simulink model "SCR_SiLS2"  (R2021b)
settings: Solver=FixedStepDiscrete  StartTime=0.0  StopTime=inf  FixedStep=0.001  RelTol=1e-3
model workspace (MAT data in the model file):
  DataSet = []
  DebugLevel = 0
  GuiObj = 0
  GuiObjTemp = 0
  GuiPrefs.ColVis = [1 1 1 1 1 1 1 1 1 0]
  GuiPrefs.Mode = 0
  GuiPrefs.View = 1
  GuiPrefs.Hierarchy = 1
  GuiPrefs.BatchMode = 0
  GuiPrefs.ConsistentAccess = 0
  M1TargetParameters.TargetIp = '192.168.0.153'
  M1TargetParameters.M1ControllerName = 'M1Controller'
  M1TargetParameters.SwModuleName = 'SILS'
  M1TargetParameters.ApplPartition = 2
  M1TargetParameters.BasePriority = 30
  M1TargetParameters.CoreCategory = ''
  M1TargetParameters.DownlToM1Contr = 'on'
  M1TargetParameters.PermanentInstall = 'on'
  M1TargetParameters.DeviceOnM1 = 'Application path'
  M1TargetParameters.SendEOI = 'on'
  M1TargetParameters.ControllerUsr = 'M1'
  M1TargetParameters.ControllerPwd = 'bachmann'
  M1TargetParameters.ModDebugLevel = '0x0'
  NbrOfParams = 0
  NbrOfRem = 0
  save_DataSet = []
  save_NbrOfParams = 0
  save_NbrOfRem = 0
undefined symbols (not defined in the file or in its folder): AI_Test1, AO_Test1, NONOXR4, PLC_PRG, var1_INT16_LREAL_scalar_bus_200_mixed_aligned_out, X20I0Mat_typ, X20IOMat, X20IOSim
libraries: bur_blks x62, M1SWBlocks x11, simulink x1
(part 1 of 2)
CloseFcn:
  | ModelCloseCallback(gcs, 'FigureName', 'M1DownloadSettings');
  | ModelCloseCallback(gcs, 'FigureName', 'SourceInclusion');
settings Model: ExtModeSkipDownloadWhenConnect=on  Creator=gione  LastModifiedBy=gione
settings HardwareCC: ProdBitPerPointer=32  ProdBitPerSizeT=32  ProdBitPerPtrDiffT=32  ProdLargestAtomicInteger=Long  ProdWordSize=32  ProdLongLongMode=on  ProdHWDeviceType=Bachmann->Bachmann M1 Controller  TargetLargestAtomicInteger=Long  TargetLargestAtomicFloat=Float  TargetLongLongMode=on  TargetIntDivRoundTo=Zero  TargetEndianess=LittleEndian  TargetHWDeviceType=Bachmann->Bachmann M1 Controller  ProdEqTarget=off
settings RTWCC: Description=Bachmann M1 SW Module Creator  SystemTargetFile=m1target.tlc  TemplateMakefile=m1target.tmf  GenerateReport=on  LaunchReport=on
settings STFCustomTargetCC: SystemTargetFile=m1target.tlc
settings GRTTargetCC: TargetLangStandard=C89/C90 (ANSI)  ParMdlRefBuildCompliant=off  CompOptLevelCompliant=off  ConcurrentExecutionCompliant=off  CombineOutputUpdateFcns=off  MatFileLogging=off  CPPClassGenCompliant=off  GRTInterface=on  UseToolchainInfoCompliant=off  ExtMode=on  ExtModeMexFile=ext_m1target_comm  ExtModeMexArgs='192.168.0.153' 0 17725 'SILS' 'M1' 'bachmann'

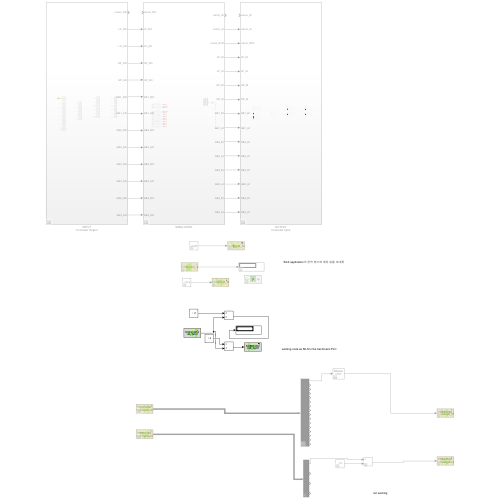
[thumbnail: Simulink's stored preview of the top-level diagram]
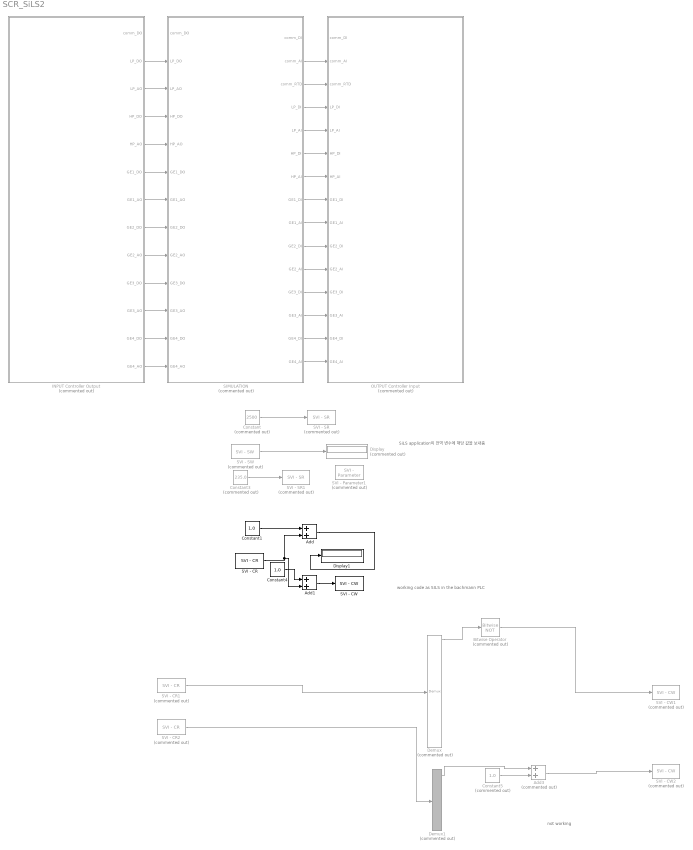
== system SCR_SiLS2 ==
  note: SiLS application의 전역 변수에 해당 값을 보내줌
  note: working code as SILS in the bachmann PLC
  note: not working
  Add : Sum
  Add1 : Sum
  Add3 : Sum  Commented=on
  Bitwise Operator : simulink/Logic and Bit Operations/Bitwise Operator  Commented=on  logicop=NOT  UseBitMask=off  BitMask=bin2dec('11011001')  BitMaskRealWorld=Stored Integer
  Constant : Constant  Commented=on  Value=2500
  Constant1 : Constant  Value=1.0
  Constant3 : Constant  Commented=on  Value=235.0
      settings: CopyFcn=CopyBlockEntries(gcs, gcb, 'Constant3');  DeleteFcn=RefreshFile(gcs, gcb, 1);  NameChangeFcn=RefreshFile(gcs, gcb, 0);
  Constant4 : Constant  Value=1.0
  Constant5 : Constant  Commented=on  Value=1.0
  Demux : Demux  Commented=on  Outputs=16  BusSelectionMode=on
  Demux1 : Demux  Commented=on  BusSelectionMode=on
  Display : Display  Commented=on
  Display1 : Display
  INPUT Controller Output : Subsystem  Commented=on
  OUTPUT Controller Input : Subsystem  Commented=on
  SIMULATION : Subsystem  Commented=on
  SVI - CR : M1SWBlocks/SVI Blocks/SVI - CR  Description=SVI client read block  svi_taskname=NONOXR4  svi_varname=.AI_Test1  svi_datatype=double  svi_retcodeoutput=off  svi_enablesettrigger=off  svi_settrigger=rising  svi_reconnect=off  svi_valdurlostconn=Last value  svi_valueinternal=567657567567  svi_sampletime=0.001  svi_simavailable=off  svi_roundtype=Zero
      settings: SourceProductName=Bachmann M1 Software
  SVI - CR1 : M1SWBlocks/SVI Blocks/SVI - CR  Description=SVI client read block  Commented=on  svi_taskname=NONOXR4  svi_varname=.IOSim/Comm/DI_0  svi_datatype=Bus: DO_Value  svi_retcodeoutput=off  svi_enablesettrigger=off  svi_settrigger=rising  svi_reconnect=off  svi_valdurlostconn=Last value  svi_valueinternal=567657567567  svi_sampletime=Ts_com  svi_simavailable=off  svi_roundtype=Zero
      settings: SourceProductName=Bachmann M1 Software
  SVI - CR2 : M1SWBlocks/SVI Blocks/SVI - CR  Description=SVI client read block  Commented=on  svi_taskname=NONOXR4  svi_varname=.IOSim/Comm/AO_0  svi_datatype=Bus: AO_Value  svi_retcodeoutput=off  svi_enablesettrigger=off  svi_settrigger=rising  svi_reconnect=off  svi_valdurlostconn=Last value  svi_valueinternal=567657567567  svi_sampletime=Ts_com  svi_simavailable=off  svi_roundtype=Zero
      settings: SourceProductName=Bachmann M1 Software
  SVI - CW : M1SWBlocks/SVI Blocks/SVI - CW  Description=SVI client write block  svi_taskname=NONOXR4  svi_varname=.AO_Test1  svi_datatype=double  svi_roundtype=Zero  svi_retcodeoutput=off  svi_enablesettrigger=off  svi_settrigger=rising  svi_reconnect=off  svi_simavailable=off
      settings: SourceProductName=Bachmann M1 Software
  SVI - CW1 : M1SWBlocks/SVI Blocks/SVI - CW  Description=SVI client write block  Commented=on  svi_taskname=NONOXR4  svi_varname='.IOSim/Comm/DI_0/Value0'  svi_datatype=boolean  svi_roundtype=Zero  svi_retcodeoutput=off  svi_enablesettrigger=off  svi_settrigger=rising  svi_reconnect=off  svi_simavailable=off
      settings: SourceProductName=Bachmann M1 Software
  SVI - CW2 : M1SWBlocks/SVI Blocks/SVI - CW  Description=SVI client write block  Commented=on  svi_taskname=NONOXR4  svi_varname='NONOXR4/.IOSim/Comm/AI_0/Value0'  svi_datatype=single  svi_roundtype=Zero  svi_retcodeoutput=off  svi_enablesettrigger=off  svi_settrigger=rising  svi_reconnect=off  svi_simavailable=off
      settings: SourceProductName=Bachmann M1 Software
  SVI - Parameter1 : M1SWBlocks/SVI Blocks/SVI - Parameter  Commented=on  svi_changeCount=1
      settings: SourceProductName=Bachmann M1 Software
  SVI - SR : M1SWBlocks/SVI Blocks/SVI - SR  Description=SVI server readonly block  Commented=on  svi_name=NONOXR4/AI_Test1  svi_modelname=off  svi_subsysname=off  svi_datatype=Inherit: auto  svi_alignment=4 bytes aligned  svi_roundtype=Nearest  svi_consistent=off  svi_simavailable=off
      settings: SourceProductName=Bachmann M1 Software
  SVI - SR1 : M1SWBlocks/SVI Blocks/SVI - SR  Description=SVI server readonly block  Commented=on  svi_name=NONOXR4/AI_Test1  svi_modelname=off  svi_subsysname=off  svi_datatype=Inherit: auto  svi_alignment=4 bytes aligned  svi_roundtype=Nearest  svi_consistent=off  svi_simavailable=off
      settings: SourceProductName=Bachmann M1 Software
  SVI - SW : M1SWBlocks/SVI Blocks/SVI - SW  Description=SVI server read/write block  Commented=on  svi_name=NONOXR4/AO_Test1  svi_modelname=off  svi_subsysname=off  svi_initvalue=0  svi_datatype=Inherit: Inherit via back propagation  svi_alignment=4 bytes aligned  svi_varremanent=off  svi_consistent=on  svi_sampletime=-1  svi_simavailable=off  svi_roundtype=Zero
      settings: SourceProductName=Bachmann M1 Software
  wires:
  Constant/1 -> SVI - SR/1
  SVI - SW/1 -> Display/1
  Constant1/1 -> Add/1
  SVI - CR/1 -> Add1/2, Add/2
  Add/1 -> Display1/1
  Constant3/1 -> SVI - SR1/1
  Constant4/1 -> Add1/1
  Add1/1 -> SVI - CW/1
  SIMULATION/15(GE4_AI) -> OUTPUT Controller Input/15(GE4_AI)
  SIMULATION/14(GE4_DI) -> OUTPUT Controller Input/14(GE4_DI)
  SIMULATION/11(GE2_AI) -> OUTPUT Controller Input/11(GE2_AI)
  SIMULATION/4(LP_DI) -> OUTPUT Controller Input/4(LP_DI)
  SIMULATION/5(LP_AI) -> OUTPUT Controller Input/5(LP_AI)
  INPUT Controller Output/9(GE2_AO) -> SIMULATION/9(GE2_AO)
  INPUT Controller Output/10(GE3_DO) -> SIMULATION/10(GE3_DO)
  INPUT Controller Output/7(GE1_AO) -> SIMULATION/7(GE1_AO)
  INPUT Controller Output/8(GE2_DO) -> SIMULATION/8(GE2_DO)
  INPUT Controller Output/6(GE1_DO) -> SIMULATION/6(GE1_DO)
  INPUT Controller Output/3(LP_AO) -> SIMULATION/3(LP_AO)
  INPUT Controller Output/4(HP_DO) -> SIMULATION/4(HP_DO)
  SIMULATION/2(comm_AI) -> OUTPUT Controller Input/2(comm_AI)
  SIMULATION/8(GE1_DI) -> OUTPUT Controller Input/8(GE1_DI)
  INPUT Controller Output/5(HP_AO) -> SIMULATION/5(HP_AO)
  INPUT Controller Output/2(LP_DO) -> SIMULATION/2(LP_DO)
  SIMULATION/6(HP_DI) -> OUTPUT Controller Input/6(HP_DI)
  SIMULATION/13(GE3_AI) -> OUTPUT Controller Input/13(GE3_AI)
  SIMULATION/9(GE1_AI) -> OUTPUT Controller Input/9(GE1_AI)
  SIMULATION/3(comm_RTD) -> OUTPUT Controller Input/3(comm_RTD)
  INPUT Controller Output/13(GE4_AO) -> SIMULATION/13(GE4_AO)
  INPUT Controller Output/12(GE4_DO) -> SIMULATION/12(GE4_DO)
  INPUT Controller Output/11(GE3_AO) -> SIMULATION/11(GE3_AO)
  SIMULATION/7(HP_AI) -> OUTPUT Controller Input/7(HP_AI)
  SIMULATION/12(GE3_DI) -> OUTPUT Controller Input/12(GE3_DI)
  SIMULATION/10(GE2_DI) -> OUTPUT Controller Input/10(GE2_DI)
  SVI - CR1/1 -> Demux/1
  Demux/1 -> Bitwise Operator/1
  SVI - CR2/1 -> Demux1/1
  Demux1/1 -> Add3/1
  Add3/1 -> SVI - CW2/1
  Bitwise Operator/1 -> SVI - CW1/1
  Constant5/1 -> Add3/2

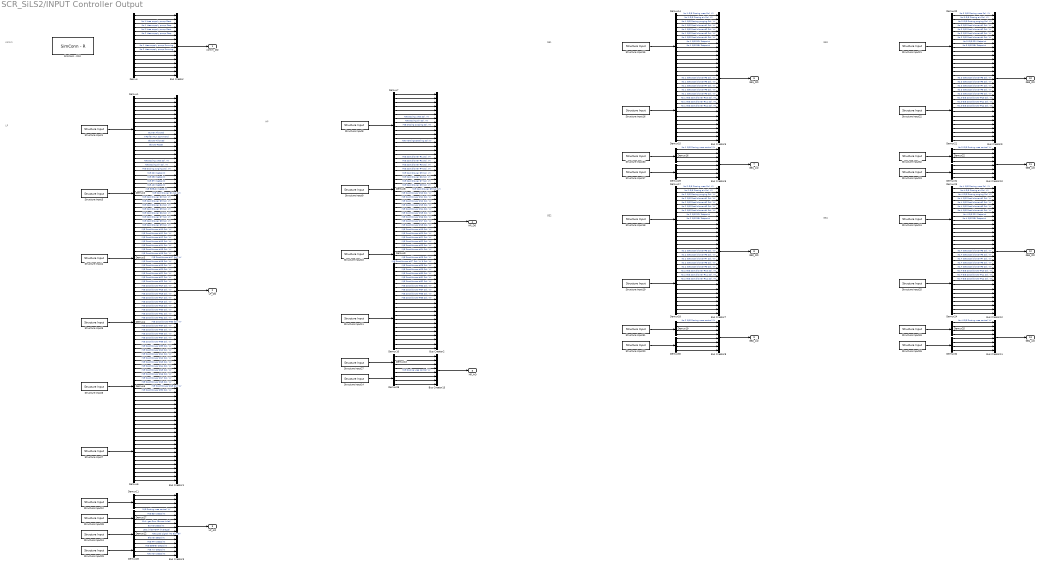
== system SCR_SiLS2/INPUT Controller Output ==
  note: comm
  note: LP
  note: HP
  note: GE1
  note: GE2
  note: GE3
  note: GE4
  Bus Creator : BusCreator  Inputs=16
  Bus Creator1 : BusCreator  Inputs=96
  Bus Creator{6,8,10..11,13} (5 alike) : BusCreator  Inputs=8
  Bus Creator{5,7,9,12} (4 alike) : BusCreator  Inputs=32
  Bus Creator2 : BusCreator  Inputs=64
  Bus Creator3 : BusCreator  Inputs=16
  Demux{,1..10,14..15,17..18,20..21,23..24} (19 alike) : Demux  Outputs=16
  Demux{11..13,16,19,22,25..32} (14 alike) : Demux
  SimConn - R10 : M1SWBlocks/SimConn Blocks/SimConn - R  connVarName=ConnVar  InswModuleName='NONOXR4'  swModuleName=PLC_DSRC  InvarName='.X20IOSim.Comm.DOF322[0].Value'  varName=PLC_PRG/var1_INT16_LREAL_scalar_bus_200_mixed_aligned_out  varDataType=Inherit: Inherit via back propagation  enRetOutput=on  enGetTrigger=off  getTrigger=rising  valDurLostConn=Zero  internalVal=0  DataDim=1  enSampTimMon=on  sampleTime=Ts_com
      settings: SourceProductName=Bachmann M1 Software
  Structure Input1 : bur_blks/Structure Input  Tag=GLOBAL BOOL X20IOSim.LP.DOF322[0].Value [0...15]  bur_var_name=X20IOSim.LP.DOF322[0].Value  bur_scope=GLOBAL  bur_struct_name=X20IOSim  bur_data_type=BOOL  bur_array_index=15  bur_data_type_num=8  bur_AS_string=X20IOSim : X20I0Mat_typ := (0); (**)  bur_struct_reference=X20I0Mat_typ.LP.DOF322(0).Value  bur_memory=standard
      settings: AttributesFormatString=%<Tag>  SourceProductName=B&R Automation Studio Toolbox
  Structure Input10 : bur_blks/Structure Input  Tag=GLOBAL BOOL X20IOSim.HP.DOF322[2].Value [0...15]  bur_var_name=X20IOSim.HP.DOF322[2].Value  bur_scope=GLOBAL  bur_struct_name=X20IOSim  bur_data_type=BOOL  bur_array_index=15  bur_data_type_num=8  bur_AS_string=X20IOSim : X20I0Mat_typ := (0); (**)  bur_struct_reference=X20I0Mat_typ.HP.DOF322(2).Value  bur_memory=standard
      settings: AttributesFormatString=%<Tag>  SourceProductName=B&R Automation Studio Toolbox
  Structure Input11 : bur_blks/Structure Input  Tag=GLOBAL BOOL X20IOSim.HP.DOF322[3].Value [0...15]  bur_var_name=X20IOSim.HP.DOF322[3].Value  bur_scope=GLOBAL  bur_struct_name=X20IOSim  bur_data_type=BOOL  bur_array_index=15  bur_data_type_num=8  bur_AS_string=X20IOSim : X20I0Mat_typ := (0); (**)  bur_struct_reference=X20I0Mat_typ.HP.DOF322(3).Value  bur_memory=standard
      settings: AttributesFormatString=%<Tag>  SourceProductName=B&R Automation Studio Toolbox
  Structure Input12 : bur_blks/Structure Input  Tag=GLOBAL REAL X20IOSim.LP.AO4622[0].Value [0...3]  bur_var_name=X20IOSim.LP.AO4622[0].Value  bur_scope=GLOBAL  bur_struct_name=X20IOSim  bur_data_type=REAL  bur_array_index=3  bur_data_type_num=1  bur_AS_string=X20IOSim : X20I0Mat_typ := (0); (**)  bur_struct_reference=X20I0Mat_typ.LP.AO4622(0).Value  bur_memory=standard
      settings: AttributesFormatString=%<Tag>  SourceProductName=B&R Automation Studio Toolbox
  Structure Input13 : bur_blks/Structure Input  Tag=GLOBAL REAL X20IOSim.LP.AO4622[2].Value [0...3]  bur_var_name=X20IOSim.LP.AO4622[2].Value  bur_scope=GLOBAL  bur_struct_name=X20IOSim  bur_data_type=REAL  bur_array_index=3  bur_data_type_num=1  bur_AS_string=X20IOSim : X20I0Mat_typ := (0); (**)  bur_struct_reference=X20I0Mat_typ.LP.AO4622(2).Value  bur_memory=standard
      settings: AttributesFormatString=%<Tag>  SourceProductName=B&R Automation Studio Toolbox
  Structure Input14 : bur_blks/Structure Input  Tag=GLOBAL REAL X20IOSim.HP.AO4622[1].Value [0...3]  bur_var_name=X20IOSim.HP.AO4622[1].Value  bur_scope=GLOBAL  bur_struct_name=X20IOSim  bur_data_type=REAL  bur_array_index=3  bur_data_type_num=1  bur_AS_string=X20IOSim : X20I0Mat_typ := (0); (**)  bur_struct_reference=X20I0Mat_typ.HP.AO4622(1).Value  bur_memory=standard
      settings: AttributesFormatString=%<Tag>  SourceProductName=B&R Automation Studio Toolbox
  Structure Input15 : bur_blks/Structure Input  Tag=GLOBAL BOOL X20IOSim.GE1.DOF322[0].Value [0...15]  bur_var_name=X20IOSim.GE1.DOF322[0].Value  bur_scope=GLOBAL  bur_struct_name=X20IOSim  bur_data_type=BOOL  bur_array_index=15  bur_data_type_num=8  bur_AS_string=X20IOSim : X20I0Mat_typ := (0); (**)  bur_struct_reference=X20I0Mat_typ.GE1.DOF322(0).Value  bur_memory=standard
      settings: AttributesFormatString=%<Tag>  SourceProductName=B&R Automation Studio Toolbox
  Structure Input16 : bur_blks/Structure Input  Tag=GLOBAL BOOL X20IOSim.GE1.DOF322[1].Value [0...15]  bur_var_name=X20IOSim.GE1.DOF322[1].Value  bur_scope=GLOBAL  bur_struct_name=X20IOSim  bur_data_type=BOOL  bur_array_index=15  bur_data_type_num=8  bur_AS_string=X20IOSim : X20I0Mat_typ := (0); (**)  bur_struct_reference=X20I0Mat_typ.GE1.DOF322(1).Value  bur_memory=standard
      settings: AttributesFormatString=%<Tag>  SourceProductName=B&R Automation Studio Toolbox
  Structure Input17 : bur_blks/Structure Input  Tag=GLOBAL REAL X20IOSim.GE1.AO4622[1].Value [0...3]  bur_var_name=X20IOSim.GE1.AO4622[1].Value  bur_scope=GLOBAL  bur_struct_name=X20IOSim  bur_data_type=REAL  bur_array_index=3  bur_data_type_num=1  bur_AS_string=X20IOSim : X20I0Mat_typ := (0); (**)  bur_struct_reference=X20I0Mat_typ.GE1.AO4622(1).Value  bur_memory=standard
      settings: AttributesFormatString=%<Tag>  SourceProductName=B&R Automation Studio Toolbox
  Structure Input18 : bur_blks/Structure Input  Tag=GLOBAL BOOL X20IOSim.GE2.DOF322[0].Value [0...15]  bur_var_name=X20IOSim.GE2.DOF322[0].Value  bur_scope=GLOBAL  bur_struct_name=X20IOSim  bur_data_type=BOOL  bur_array_index=15  bur_data_type_num=8  bur_AS_string=X20IOSim : X20I0Mat_typ := (0); (**)  bur_struct_reference=X20I0Mat_typ.GE2.DOF322(0).Value  bur_memory=standard
      settings: AttributesFormatString=%<Tag>  SourceProductName=B&R Automation Studio Toolbox
  Structure Input19 : bur_blks/Structure Input  Tag=GLOBAL BOOL X20IOSim.GE2.DOF322[1].Value [0...15]  bur_var_name=X20IOSim.GE2.DOF322[1].Value  bur_scope=GLOBAL  bur_struct_name=X20IOSim  bur_data_type=BOOL  bur_array_index=15  bur_data_type_num=8  bur_AS_string=X20IOSim : X20I0Mat_typ := (0); (**)  bur_struct_reference=X20I0Mat_typ.GE2.DOF322(1).Value  bur_memory=standard
      settings: AttributesFormatString=%<Tag>  SourceProductName=B&R Automation Studio Toolbox
  Structure Input20 : bur_blks/Structure Input  Tag=GLOBAL REAL X20IOSim.GE2.AO4622[1].Value [0...3]  bur_var_name=X20IOSim.GE2.AO4622[1].Value  bur_scope=GLOBAL  bur_struct_name=X20IOSim  bur_data_type=REAL  bur_array_index=3  bur_data_type_num=1  bur_AS_string=X20IOSim : X20I0Mat_typ := (0); (**)  bur_struct_reference=X20I0Mat_typ.GE2.AO4622(1).Value  bur_memory=standard
      settings: AttributesFormatString=%<Tag>  SourceProductName=B&R Automation Studio Toolbox
  Structure Input21 : bur_blks/Structure Input  Tag=GLOBAL BOOL X20IOSim.GE3.DOF322[0].Value [0...15]  bur_var_name=X20IOSim.GE3.DOF322[0].Value  bur_scope=GLOBAL  bur_struct_name=X20IOSim  bur_data_type=BOOL  bur_array_index=15  bur_data_type_num=8  bur_AS_string=X20IOSim : X20I0Mat_typ := (0); (**)  bur_struct_reference=X20I0Mat_typ.GE3.DOF322(0).Value  bur_memory=standard
      settings: AttributesFormatString=%<Tag>  SourceProductName=B&R Automation Studio Toolbox
  Structure Input22 : bur_blks/Structure Input  Tag=GLOBAL BOOL X20IOSim.GE3.DOF322[1].Value [0...15]  bur_var_name=X20IOSim.GE3.DOF322[1].Value  bur_scope=GLOBAL  bur_struct_name=X20IOSim  bur_data_type=BOOL  bur_array_index=15  bur_data_type_num=8  bur_AS_string=X20IOSim : X20I0Mat_typ := (0); (**)  bur_struct_reference=X20I0Mat_typ.GE3.DOF322(1).Value  bur_memory=standard
      settings: AttributesFormatString=%<Tag>  SourceProductName=B&R Automation Studio Toolbox
  Structure Input23 : bur_blks/Structure Input  Tag=GLOBAL REAL X20IOSim.GE3.AO4622[1].Value [0...3]  bur_var_name=X20IOSim.GE3.AO4622[1].Value  bur_scope=GLOBAL  bur_struct_name=X20IOSim  bur_data_type=REAL  bur_array_index=3  bur_data_type_num=1  bur_AS_string=X20IOSim : X20I0Mat_typ := (0); (**)  bur_struct_reference=X20I0Mat_typ.GE3.AO4622(1).Value  bur_memory=standard
      settings: AttributesFormatString=%<Tag>  SourceProductName=B&R Automation Studio Toolbox
  Structure Input24 : bur_blks/Structure Input  Tag=GLOBAL BOOL X20IOSim.GE4.DOF322[0].Value [0...15]  bur_var_name=X20IOSim.GE4.DOF322[0].Value  bur_scope=GLOBAL  bur_struct_name=X20IOSim  bur_data_type=BOOL  bur_array_index=15  bur_data_type_num=8  bur_AS_string=X20IOSim : X20I0Mat_typ := (0); (**)  bur_struct_reference=X20I0Mat_typ.GE4.DOF322(0).Value  bur_memory=standard
      settings: AttributesFormatString=%<Tag>  SourceProductName=B&R Automation Studio Toolbox
  Structure Input25 : bur_blks/Structure Input  Tag=GLOBAL BOOL X20IOSim.GE4.DOF322[1].Value [0...15]  bur_var_name=X20IOSim.GE4.DOF322[1].Value  bur_scope=GLOBAL  bur_struct_name=X20IOSim  bur_data_type=BOOL  bur_array_index=15  bur_data_type_num=8  bur_AS_string=X20IOSim : X20I0Mat_typ := (0); (**)  bur_struct_reference=X20I0Mat_typ.GE4.DOF322(1).Value  bur_memory=standard
      settings: AttributesFormatString=%<Tag>  SourceProductName=B&R Automation Studio Toolbox
  Structure Input26 : bur_blks/Structure Input  Tag=GLOBAL REAL X20IOSim.GE4.AO4622[1].Value [0...3]  bur_var_name=X20IOSim.GE4.AO4622[1].Value  bur_scope=GLOBAL  bur_struct_name=X20IOSim  bur_data_type=REAL  bur_array_index=3  bur_data_type_num=1  bur_AS_string=X20IOSim : X20I0Mat_typ := (0); (**)  bur_struct_reference=X20I0Mat_typ.GE4.AO4622(1).Value  bur_memory=standard
      settings: AttributesFormatString=%<Tag>  SourceProductName=B&R Automation Studio Toolbox
  Structure Input27 : bur_blks/Structure Input  Tag=GLOBAL REAL X20IOSim.HP.AO4622[0].Value [0...3]  bur_var_name=X20IOSim.HP.AO4622[0].Value  bur_scope=GLOBAL  bur_struct_name=X20IOSim  bur_data_type=REAL  bur_array_index=3  bur_data_type_num=1  bur_AS_string=X20IOSim : X20I0Mat_typ := (0); (**)  bur_struct_reference=X20I0Mat_typ.HP.AO4622(0).Value  bur_memory=standard
      settings: AttributesFormatString=%<Tag>  SourceProductName=B&R Automation Studio Toolbox
  Structure Input28 : bur_blks/Structure Input  Tag=GLOBAL REAL X20IOSim.LP.AO4622[1].Value [0...3]  bur_var_name=X20IOSim.LP.AO4622[1].Value  bur_scope=GLOBAL  bur_struct_name=X20IOSim  bur_data_type=REAL  bur_array_index=3  bur_data_type_num=1  bur_AS_string=X20IOSim : X20I0Mat_typ := (0); (**)  bur_struct_reference=X20I0Mat_typ.LP.AO4622(1).Value  bur_memory=standard
      settings: AttributesFormatString=%<Tag>  SourceProductName=B&R Automation Studio Toolbox
  Structure Input29 : bur_blks/Structure Input  Tag=GLOBAL REAL X20IOSim.LP.AO4622[3].Value [0...3]  bur_var_name=X20IOSim.LP.AO4622[3].Value  bur_scope=GLOBAL  bur_struct_name=X20IOSim  bur_data_type=REAL  bur_array_index=3  bur_data_type_num=1  bur_AS_string=X20IOSim : X20I0Mat_typ := (0); (**)  bur_struct_reference=X20I0Mat_typ.LP.AO4622(3).Value  bur_memory=standard
      settings: AttributesFormatString=%<Tag>  SourceProductName=B&R Automation Studio Toolbox
  Structure Input3 : bur_blks/Structure Input  Tag=GLOBAL BOOL X20IOSim.LP.DOF322[1].Value [0...15]  bur_var_name=X20IOSim.LP.DOF322[1].Value  bur_scope=GLOBAL  bur_struct_name=X20IOSim  bur_data_type=BOOL  bur_array_index=15  bur_data_type_num=8  bur_AS_string=X20IOSim : X20I0Mat_typ := (0); (**)  bur_struct_reference=X20I0Mat_typ.LP.DOF322(1).Value  bur_memory=standard
      settings: AttributesFormatString=%<Tag>  SourceProductName=B&R Automation Studio Toolbox
  Structure Input30 : bur_blks/Structure Input  Tag=GLOBAL REAL X20IOSim.GE1.AO4622[0].Value [0...3]  bur_var_name=X20IOSim.GE1.AO4622[0].Value  bur_scope=GLOBAL  bur_struct_name=X20IOSim  bur_data_type=REAL  bur_array_index=3  bur_data_type_num=1  bur_AS_string=X20IOSim : X20I0Mat_typ := (0); (**)  bur_struct_reference=X20I0Mat_typ.GE1.AO4622(0).Value  bur_memory=standard
      settings: AttributesFormatString=%<Tag>  SourceProductName=B&R Automation Studio Toolbox
  Structure Input31 : bur_blks/Structure Input  Tag=GLOBAL REAL X20IOSim.GE2.AO4622[0].Value [0...3]  bur_var_name=X20IOSim.GE2.AO4622[0].Value  bur_scope=GLOBAL  bur_struct_name=X20IOSim  bur_data_type=REAL  bur_array_index=3  bur_data_type_num=1  bur_AS_string=X20IOSim : X20I0Mat_typ := (0); (**)  bur_struct_reference=X20I0Mat_typ.GE2.AO4622(0).Value  bur_memory=standard
      settings: AttributesFormatString=%<Tag>  SourceProductName=B&R Automation Studio Toolbox
  Structure Input32 : bur_blks/Structure Input  Tag=GLOBAL REAL X20IOSim.GE3.AO4622[0].Value [0...3]  bur_var_name=X20IOSim.GE3.AO4622[0].Value  bur_scope=GLOBAL  bur_struct_name=X20IOSim  bur_data_type=REAL  bur_array_index=3  bur_data_type_num=1  bur_AS_string=X20IOSim : X20I0Mat_typ := (0); (**)  bur_struct_reference=X20I0Mat_typ.GE3.AO4622(0).Value  bur_memory=standard
      settings: AttributesFormatString=%<Tag>  SourceProductName=B&R Automation Studio Toolbox
  Structure Input33 : bur_blks/Structure Input  Tag=GLOBAL REAL X20IOSim.GE4.AO4622[0].Value [0...3]  bur_var_name=X20IOSim.GE4.AO4622[0].Value  bur_scope=GLOBAL  bur_struct_name=X20IOSim  bur_data_type=REAL  bur_array_index=3  bur_data_type_num=1  bur_AS_string=X20IOSim : X20I0Mat_typ := (0); (**)  bur_struct_reference=X20I0Mat_typ.GE4.AO4622(0).Value  bur_memory=standard
      settings: AttributesFormatString=%<Tag>  SourceProductName=B&R Automation Studio Toolbox
  Structure Input4 : bur_blks/Structure Input  Tag=GLOBAL BOOL X20IOSim.LP.DOF322[2].Value [0...15]  bur_var_name=X20IOSim.LP.DOF322[2].Value  bur_scope=GLOBAL  bur_struct_name=X20IOSim  bur_data_type=BOOL  bur_array_index=15  bur_data_type_num=8  bur_AS_string=X20IOSim : X20I0Mat_typ := (0); (**)  bur_struct_reference=X20I0Mat_typ.LP.DOF322(2).Value  bur_memory=standard
      settings: AttributesFormatString=%<Tag>  SourceProductName=B&R Automation Studio Toolbox
  Structure Input5 : bur_blks/Structure Input  Tag=GLOBAL BOOL X20IOSim.LP.DOF322[3].Value [0...15]  bur_var_name=X20IOSim.LP.DOF322[3].Value  bur_scope=GLOBAL  bur_struct_name=X20IOSim  bur_data_type=BOOL  bur_array_index=15  bur_data_type_num=8  bur_AS_string=X20IOSim : X20I0Mat_typ := (0); (**)  bur_struct_reference=X20I0Mat_typ.LP.DOF322(3).Value  bur_memory=standard
      settings: AttributesFormatString=%<Tag>  SourceProductName=B&R Automation Studio Toolbox
  Structure Input6 : bur_blks/Structure Input  Tag=GLOBAL BOOL X20IOSim.LP.DOF322[4].Value [0...15]  bur_var_name=X20IOSim.LP.DOF322[4].Value  bur_scope=GLOBAL  bur_struct_name=X20IOSim  bur_data_type=BOOL  bur_array_index=15  bur_data_type_num=8  bur_AS_string=X20IOSim : X20I0Mat_typ := (0); (**)  bur_struct_reference=X20I0Mat_typ.LP.DOF322(4).Value  bur_memory=standard
      settings: AttributesFormatString=%<Tag>  SourceProductName=B&R Automation Studio Toolbox
  Structure Input7 : bur_blks/Structure Input  Tag=GLOBAL BOOL X20IOSim.LP.DOF322[5].Value [0...15]  bur_var_name=X20IOSim.LP.DOF322[5].Value  bur_scope=GLOBAL  bur_struct_name=X20IOSim  bur_data_type=BOOL  bur_array_index=15  bur_data_type_num=8  bur_AS_string=X20IOSim : X20I0Mat_typ := (0); (**)  bur_struct_reference=X20I0Mat_typ.LP.DOF322(5).Value  bur_memory=standard
      settings: AttributesFormatString=%<Tag>  SourceProductName=B&R Automation Studio Toolbox
  Structure Input8 : bur_blks/Structure Input  Tag=GLOBAL BOOL X20IOSim.HP.DOF322[0].Value [0...15]  bur_var_name=X20IOSim.HP.DOF322[0].Value  bur_scope=GLOBAL  bur_struct_name=X20IOSim  bur_data_type=BOOL  bur_array_index=15  bur_data_type_num=8  bur_AS_string=X20IOSim : X20I0Mat_typ := (0); (**)  bur_struct_reference=X20I0Mat_typ.HP.DOF322(0).Value  bur_memory=standard
      settings: AttributesFormatString=%<Tag>  SourceProductName=B&R Automation Studio Toolbox
  Structure Input9 : bur_blks/Structure Input  Tag=GLOBAL BOOL X20IOSim.HP.DOF322[1].Value [0...15]  bur_var_name=X20IOSim.HP.DOF322[1].Value  bur_scope=GLOBAL  bur_struct_name=X20IOSim  bur_data_type=BOOL  bur_array_index=15  bur_data_type_num=8  bur_AS_string=X20IOSim : X20I0Mat_typ := (0); (**)  bur_struct_reference=X20I0Mat_typ.HP.DOF322(1).Value  bur_memory=standard
      settings: AttributesFormatString=%<Tag>  SourceProductName=B&R Automation Studio Toolbox
  comm_DO : Outport  VectorParamsAs1DForOutWhenUnconnected=off
  LP_DO : Outport  Port=2  VectorParamsAs1DForOutWhenUnconnected=off
  LP_AO : Outport  Port=3  VectorParamsAs1DForOutWhenUnconnected=off
  HP_DO : Outport  Port=4  VectorParamsAs1DForOutWhenUnconnected=off
  HP_AO : Outport  Port=5  VectorParamsAs1DForOutWhenUnconnected=off
  GE1_DO : Outport  Port=6  VectorParamsAs1DForOutWhenUnconnected=off
  GE1_AO : Outport  Port=7  VectorParamsAs1DForOutWhenUnconnected=off
  GE2_DO : Outport  Port=8  VectorParamsAs1DForOutWhenUnconnected=off
  GE2_AO : Outport  Port=9  VectorParamsAs1DForOutWhenUnconnected=off
  GE3_DO : Outport  Port=10  VectorParamsAs1DForOutWhenUnconnected=off
  GE3_AO : Outport  Port=11  VectorParamsAs1DForOutWhenUnconnected=off
  GE4_DO : Outport  Port=12  VectorParamsAs1DForOutWhenUnconnected=off
  GE4_AO : Outport  Port=13  VectorParamsAs1DForOutWhenUnconnected=off
  wires:
  Demux17/11 -> Bus Creator7/11
  Demux10/14 -> Bus Creator2/62
  Demux3/8 -> Bus Creator1/40  "M/E Soot blower #16 Sol. VV"
  Demux17/7 -> Bus Creator7/7  "No.2 G/E Soot blower #4 Sol. VV"
  Demux11/4 -> Bus Creator3/4
  Demux5/2 -> Bus Creator1/66  "M/E Soot blower #42 Sol. VV"
  Demux18/11 -> Bus Creator7/27
  Structure Input3/1 -> Demux2/1
  Demux6/10 -> Bus Creator1/90
  Demux5/10 -> Bus Creator1/74  "M/E Soot blower #50 Sol. VV"
  Demux18/6 -> Bus Creator7/22  "No.2 G/E Soot blower #10 Sol. VV"
  Demux23/1 -> Bus Creator12/1  "No.4 G/E Dosing urea Sol. VV"
  Demux27/2 -> Bus Creator3/6  "M/E BSV Setpoint"
  Demux7/9 -> Bus Creator2/9  "M/E Dosing purging Sol. VV"
  Demux2/5 -> Bus Creator1/21  "M/E RBV Setpoint"
  Demux5/3 -> Bus Creator1/67  "M/E Soot blower #43 Sol. VV"
  Demux21/9 -> Bus Creator9/25
  Demux24/4 -> Bus Creator12/20  "No.4 G/E Soot blower #8 Sol. VV"
  Demux1/14 -> Bus Creator1/14
  Demux9/9 -> Bus Creator2/41  "M/E Soot blower #25 Sol. VV"
  Demux4/12 -> Bus Creator1/60  "M/E Soot blower #36 Sol. VV"
  Demux17/8 -> Bus Creator7/8  "No.2 G/E RSV Setpoint"
  Demux14/12 -> Bus Creator5/12
  Demux2/8 -> Bus Creator1/24  "M/E EGB-SV Setpoint"
  Demux4/4 -> Bus Creator1/52  "M/E Soot blower #28 Sol. VV"
  Demux1/13 -> Bus Creator1/13  "Blower Reset"
  Demux3/10 -> Bus Creator1/42  "M/E Soot blower #18 Sol. VV"
  Demux23/14 -> Bus Creator12/14
  Demux6/13 -> Bus Creator1/93
  Demux20/13 -> Bus Creator9/13
  Demux15/1 -> Bus Creator5/17  "No.1 G/E Soot blower #5 Sol. VV"
  Demux5/4 -> Bus Creator1/68  "M/E Soot blower #44 Sol. VV"
  Demux8/14 -> Bus Creator2/30  "M/E Soot blower #14 Sol. VV"
  Demux1/5 -> Bus Creator1/5
  ? -> Demux/1
  Demux29/2 -> Bus Creator6/6
  Demux7/4 -> Bus Creator2/4
  Demux4/10 -> Bus Creator1/58  "M/E Soot blower #34 Sol. VV"
  Demux15/6 -> Bus Creator5/22  "No.1 G/E Soot blower #10 Sol. VV"
  Demux21/1 -> Bus Creator9/17  "No.3 G/E Soot blower #5 Sol. VV"
  Demux25/2 -> Bus Creator11/2
  Demux5/1 -> Bus Creator1/65  "M/E Soot blower #41 Sol. VV"
  Demux5/7 -> Bus Creator1/71  "M/E Soot blower #47 Sol. VV"
  Demux3/14 -> Bus Creator1/46  "M/E Soot blower #22 Sol. VV"
  Demux7/10 -> Bus Creator2/10
  Demux25/1 -> Bus Creator11/1  "No.4 G/E Dosing urea control VV"
  Demux17/4 -> Bus Creator7/4  "No.2 G/E Soot blower #1 Sol. VV"
  Structure Input7/1 -> Demux6/1
  Demux24/3 -> Bus Creator12/19  "No.4 G/E Soot blower #7 Sol. VV"
  Bus Creator1/1 -> LP_DO/1
  Demux5/15 -> Bus Creator1/79
  Demux5/5 -> Bus Creator1/69  "M/E Soot blower #45 Sol. VV"
  Demux8/13 -> Bus Creator2/29  "M/E Soot blower #13 Sol. VV"
  Demux2/4 -> Bus Creator1/20  "M/E RSV Setpoint"
  Demux20/1 -> Bus Creator9/1  "No.3 G/E Dosing urea Sol. VV"
  Demux5/13 -> Bus Creator1/77
  Demux21/16 -> Bus Creator9/32
  Demux9/5 -> Bus Creator2/37  "M/E Soot blower #21 Sol. VV"
  Demux3/12 -> Bus Creator1/44  "M/E Soot blower #20 Sol. VV"
  Demux6/12 -> Bus Creator1/92
  Demux5/8 -> Bus Creator1/72  "M/E Soot blower #48 Sol. VV"
  Bus Creator/1 -> comm_DO/1
  Demux14/7 -> Bus Creator5/7  "No.1 G/E Soot blower #4 Sol. VV"
  Demux17/6 -> Bus Creator7/6  "No.2 G/E Soot blower #3 Sol. VV"
  Demux15/10 -> Bus Creator5/26
  Demux23/13 -> Bus Creator12/13
  Demux8/7 -> Bus Creator2/23  "M/E Soot blower #7 Sol. VV"
  Demux5/14 -> Bus Creator1/78
  Demux2/12 -> Bus Creator1/28  "M/E Soot blower #4 Sol. VV"
  Demux/2 -> Bus Creator/2
  Demux28/3 -> Bus Creator3/15  "M/E XIV Setpoint"
  Demux18/13 -> Bus Creator7/29
  Demux10/5 -> Bus Creator2/53
  Demux8/10 -> Bus Creator2/26  "M/E Soot blower #10 Sol. VV"
  Structure Input6/1 -> Demux5/1
  Demux5/11 -> Bus Creator1/75
  Demux24/9 -> Bus Creator12/25
  Demux/1 -> Bus Creator/1
  Structure Input10/1 -> Demux9/1
  Demux20/3 -> Bus Creator9/3  "No.3 G/E Dosing purging Sol. VV"
  Demux17/9 -> Bus Creator7/9  "No.2 G/E RBV Setpoint"
  Demux20/5 -> Bus Creator9/5  "No.3 G/E Soot blower #2 Sol. VV"
  Demux17/1 -> Bus Creator7/1  "No.2 G/E Dosing urea Sol. VV"
  Demux/13 -> Bus Creator/13
  Demux20/4 -> Bus Creator9/4  "No.3 G/E Soot blower #1 Sol. VV"
  Demux23/12 -> Bus Creator12/12
  Demux17/3 -> Bus Creator7/3  "No.2 G/E Dosing purging Sol. VV"
  Demux17/5 -> Bus Creator7/5  "No.2 G/E Soot blower #2 Sol. VV"
  Demux5/16 -> Bus Creator1/80
  Demux24/16 -> Bus Creator12/32
  Demux20/14 -> Bus Creator9/14
  Demux5/12 -> Bus Creator1/76
  Demux23/5 -> Bus Creator12/5  "No.4 G/E Soot blower #2 Sol. VV"
  Demux3/16 -> Bus Creator1/48  "M/E Soot blower #24 Sol. VV"
  Demux/10 -> Bus Creator/10  "No.2 Urea supply pump Running"
  Bus Creator3/1 -> LP_AO/1
  Demux5/9 -> Bus Creator1/73  "M/E Soot blower #49 Sol. VV"
  Demux12/2 -> Bus Creator3/10  "UDC inlet TEMP (Average)"
  Demux2/3 -> Bus Creator1/19  "M/E Dosing purging Sol. VV"
  Demux5/6 -> Bus Creator1/70  "M/E Soot blower #46 Sol. VV"
  Demux17/10 -> Bus Creator7/10
  Demux3/7 -> Bus Creator1/39  "M/E Soot blower #15 Sol. VV"
  Demux9/3 -> Bus Creator2/35  "M/E Soot blower #19 Sol. VV"
  Demux17/2 -> Bus Creator7/2  "No.2 G/E Dosing air Sol. VV"
  Bus Creator5/1 -> GE1_DO/1
  Demux31/3 -> Bus Creator10/7
  Demux/7 -> Bus Creator/7
  Demux20/7 -> Bus Creator9/7  "No.3 G/E Soot blower #4 Sol. VV"
  Demux18/10 -> Bus Creator7/26
  Demux/16 -> Bus Creator/16
  Demux31/2 -> Bus Creator10/6
  Demux17/12 -> Bus Creator7/12
  Demux3/13 -> Bus Creator1/45  "M/E Soot blower #21 Sol. VV"
  Demux9/12 -> Bus Creator2/44  "M/E Soot blower #28 Sol. VV"
  Demux23/6 -> Bus Creator12/6  "No.4 G/E Soot blower #3 Sol. VV"
  Structure Input9/1 -> Demux8/1
  Demux/3 -> Bus Creator/3  "No.1 Urea supply pump Start"
  Demux4/14 -> Bus Creator1/62  "M/E Soot blower #38 Sol. VV"
  Demux2/2 -> Bus Creator1/18  "M/E Dosing air Sol. VV"
  Demux8/15 -> Bus Creator2/31  "M/E Soot blower #15 Sol. VV"
  Demux31/4 -> Bus Creator10/8
  Structure Input24/1 -> Demux23/1
  Demux/4 -> Bus Creator/4  "No.1 Urea supply pump Stop"
  Demux2/6 -> Bus Creator1/22  "M/E BTV Setpoint"
  Demux/5 -> Bus Creator/5  "No.2 Urea supply pump Start"
  Demux9/6 -> Bus Creator2/38  "M/E Soot blower #22 Sol. VV"
  Demux2/13 -> Bus Creator1/29  "M/E Soot blower #5 Sol. VV"
  Demux/6 -> Bus Creator/6  "No.2 Urea supply pump Stop"
  Demux4/11 -> Bus Creator1/59  "M/E Soot blower #35 Sol. VV"
  Demux/8 -> Bus Creator/8
  Demux14/1 -> Bus Creator5/1  "No.1 G/E Dosing urea Sol. VV"
  Demux21/7 -> Bus Creator9/23  "No.3 G/E Soot blower #11 Sol. VV"
  Demux1/16 -> Bus Creator1/16
  Structure Input4/1 -> Demux3/1
  Demux/9 -> Bus Creator/9  "No.1 Urea supply pump Running"
  Demux18/8 -> Bus Creator7/24  "No.2 G/E Soot blower #12 Sol. VV"
  Demux/15 -> Bus Creator/15
  Demux1/7 -> Bus Creator1/7
  Demux21/8 -> Bus Creator9/24  "No.3 G/E Soot blower #12 Sol. VV"
  Demux17/16 -> Bus Creator7/16
  Demux11/3 -> Bus Creator3/3
  Demux/11 -> Bus Creator/11
  Demux3/9 -> Bus Creator1/41  "M/E Soot blower #17 Sol. VV"
  Demux4/9 -> Bus Creator1/57  "M/E Soot blower #33 Sol. VV"
  Demux8/12 -> Bus Creator2/28  "M/E Soot blower #12 Sol. VV"
  Demux15/16 -> Bus Creator5/32
  Demux10/9 -> Bus Creator2/57
  Demux10/8 -> Bus Creator2/56
  Demux4/1 -> Bus Creator1/49  "M/E Soot blower #25 Sol. VV"
  Demux20/11 -> Bus Creator9/11
  Demux7/7 -> Bus Creator2/7  "M/E Dosing urea Sol. VV"
  Demux4/8 -> Bus Creator1/56  "M/E Soot blower #32 Sol. VV"
  Demux18/12 -> Bus Creator7/28
  Demux11/2 -> Bus Creator3/2
  Demux8/4 -> Bus Creator2/20  "M/E Soot blower #4 Sol. VV"
  Demux1/15 -> Bus Creator1/15
  Demux23/9 -> Bus Creator12/9  "No.4 G/E RBV Setpoint"
  Demux7/2 -> Bus Creator2/2
  Demux4/2 -> Bus Creator1/50  "M/E Soot blower #26 Sol. VV"
  Demux1/4 -> Bus Creator1/4
  Demux8/8 -> Bus Creator2/24  "M/E Soot blower #8 Sol. VV"
  Demux21/10 -> Bus Creator9/26
  Demux28/4 -> Bus Creator3/16  "M/E XOV Setpoint"
  Structure Input25/1 -> Demux24/1
  Demux21/3 -> Bus Creator9/19  "No.3 G/E Soot blower #7 Sol. VV"
  Demux2/16 -> Bus Creator1/32  "M/E Soot blower #8 Sol. VV"
  Demux1/1 -> Bus Creator1/1
  Demux18/5 -> Bus Creator7/21  "No.2 G/E Soot blower #9 Sol. VV"
  Demux1/2 -> Bus Creator1/2
  Demux2/10 -> Bus Creator1/26  "M/E Soot blower #2 Sol. VV"
  Demux3/5 -> Bus Creator1/37  "M/E Soot blower #13 Sol. VV"
  Demux2/1 -> Bus Creator1/17  "M/E Dosing urea Sol. VV"
  Demux4/3 -> Bus Creator1/51  "M/E Soot blower #27 Sol. VV"
  Demux9/16 -> Bus Creator2/48  "M/E Soot blower #32 Sol. VV"
  Demux3/2 -> Bus Creator1/34  "M/E Soot blower #10 Sol. VV"
  Demux14/4 -> Bus Creator5/4  "No.1 G/E Soot blower #1 Sol. VV"
  Demux8/2 -> Bus Creator2/18  "M/E Soot blower #2 Sol. VV"
  Demux4/6 -> Bus Creator1/54  "M/E Soot blower #30 Sol. VV"
  Demux4/5 -> Bus Creator1/53  "M/E Soot blower #29 Sol. VV"
  Structure Input18/1 -> Demux17/1
  Structure Input16/1 -> Demux15/1
  Demux4/7 -> Bus Creator1/55  "M/E Soot blower #31 Sol. VV"
  Structure Input8/1 -> Demux7/1
  Demux3/11 -> Bus Creator1/43  "M/E Soot blower #19 Sol. VV"
  Demux3/15 -> Bus Creator1/47  "M/E Soot blower #23 Sol. VV"
  Demux9/2 -> Bus Creator2/34  "M/E Soot blower #18 Sol. VV"
  Demux20/8 -> Bus Creator9/8  "No.3 G/E RSV Setpoint"
  Demux1/3 -> Bus Creator1/3
  Demux15/15 -> Bus Creator5/31
  Demux20/10 -> Bus Creator9/10
  Demux3/3 -> Bus Creator1/35  "M/E Soot blower #11 Sol. VV"
  Demux7/3 -> Bus Creator2/3
  Demux9/15 -> Bus Creator2/47  "M/E Soot blower #31 Sol. VV"
  Demux3/4 -> Bus Creator1/36  "M/E Soot blower #12 Sol. VV"
  Demux18/4 -> Bus Creator7/20  "No.2 G/E Soot blower #8 Sol. VV"
  Demux22/3 -> Bus Creator10/3
  Demux8/11 -> Bus Creator2/27  "M/E Soot blower #11 Sol. VV"
  Demux14/13 -> Bus Creator5/13
  Demux3/6 -> Bus Creator1/38  "M/E Soot blower #14 Sol. VV"
  Demux24/5 -> Bus Creator12/21  "No.4 G/E Soot blower #9 Sol. VV"
  Demux4/15 -> Bus Creator1/63  "M/E Soot blower #39 Sol. VV"
  Demux1/10 -> Bus Creator1/10  "Burner Allowed"
  Demux6/9 -> Bus Creator1/89
  Demux1/9 -> Bus Creator1/9
  Demux2/11 -> Bus Creator1/27  "M/E Soot blower #3 Sol. VV"
  Demux14/3 -> Bus Creator5/3  "No.1 G/E Dosing purging Sol. VV"
  Structure Input22/1 -> Demux21/1
  Structure Input15/1 -> Demux14/1
  Demux1/8 -> Bus Creator1/8
  Demux1/6 -> Bus Creator1/6
  Demux8/9 -> Bus Creator2/25  "M/E Soot blower #9 Sol. VV"
  Demux15/11 -> Bus Creator5/27
  Demux20/12 -> Bus Creator9/12
  Demux6/14 -> Bus Creator1/94
  Demux2/9 -> Bus Creator1/25  "M/E Soot blower #1 Sol. VV"
  Demux1/12 -> Bus Creator1/12  "Blower Allowed"
  Demux15/7 -> Bus Creator5/23  "No.1 G/E Soot blower #11 Sol. VV"
  Demux1/11 -> Bus Creator1/11  "X-FD fan Run Command"
  Demux22/2 -> Bus Creator10/2
  Demux/12 -> Bus Creator/12
  Demux/14 -> Bus Creator/14
  Demux14/6 -> Bus Creator5/6  "No.1 G/E Soot blower #3 Sol. VV"
  Demux7/14 -> Bus Creator2/14
  Demux14/2 -> Bus Creator5/2  "No.1 G/E Dosing air Sol. VV"
  Demux9/13 -> Bus Creator2/45  "M/E Soot blower #29 Sol. VV"
  Demux23/2 -> Bus Creator12/2  "No.4 G/E Dosing air Sol. VV"
  Demux17/14 -> Bus Creator7/14
  Demux14/5 -> Bus Creator5/5  "No.1 G/E Soot blower #2 Sol. VV"
  Demux22/4 -> Bus Creator10/4
  Demux18/9 -> Bus Creator7/25
  Demux14/8 -> Bus Creator5/8  "No.1 G/E RSV Setpoint"
  Demux6/16 -> Bus Creator1/96
  Demux14/9 -> Bus Creator5/9  "No.1 G/E RBV Setpoint"
  Demux14/11 -> Bus Creator5/11
  Demux14/10 -> Bus Creator5/10
  Demux14/16 -> Bus Creator5/16
  Demux28/2 -> Bus Creator3/14  "M/E EGB-BV Setpoint"
  Demux14/14 -> Bus Creator5/14
  Demux14/15 -> Bus Creator5/15
  Demux10/16 -> Bus Creator2/64
  Demux15/12 -> Bus Creator5/28
  Demux15/3 -> Bus Creator5/19  "No.1 G/E Soot blower #7 Sol. VV"
  Demux6/8 -> Bus Creator1/88
  Structure Input12/1 -> Demux11/1
  Demux15/4 -> Bus Creator5/20  "No.1 G/E Soot blower #8 Sol. VV"
  Demux4/16 -> Bus Creator1/64  "M/E Soot blower #40 Sol. VV"
  Demux30/3 -> Bus Creator8/7
  Demux15/13 -> Bus Creator5/29
  Demux16/2 -> Bus Creator6/2
  Demux23/16 -> Bus Creator12/16
  Demux15/14 -> Bus Creator5/30
  Demux15/9 -> Bus Creator5/25
  Demux6/11 -> Bus Creator1/91
  Demux6/4 -> Bus Creator1/84
  Demux9/14 -> Bus Creator2/46  "M/E Soot blower #30 Sol. VV"
  Bus Creator11/1 -> GE4_AO/1
  Demux6/6 -> Bus Creator1/86
  Demux6/7 -> Bus Creator1/87
  Demux21/6 -> Bus Creator9/22  "No.3 G/E Soot blower #10 Sol. VV"
  Demux7/1 -> Bus Creator2/1
  Demux6/2 -> Bus Creator1/82
  Demux20/16 -> Bus Creator9/16
  Demux6/1 -> Bus Creator1/81
  Demux6/5 -> Bus Creator1/85
  Demux6/3 -> Bus Creator1/83
  Demux6/15 -> Bus Creator1/95
  Demux10/6 -> Bus Creator2/54
  Demux21/13 -> Bus Creator9/29
  Demux17/13 -> Bus Creator7/13
  Demux30/2 -> Bus Creator8/6
  Demux7/13 -> Bus Creator2/13  "M/E Venting&Sealing Sol.VV"
  Demux7/8 -> Bus Creator2/8  "M/E Dosing air Sol. VV"
  Demux20/9 -> Bus Creator9/9  "No.3 G/E RBV Setpoint"
  Demux8/6 -> Bus Creator2/22  "M/E Soot blower #6 Sol. VV"
  Demux7/16 -> Bus Creator2/16
  Structure Input19/1 -> Demux18/1
  Demux31/1 -> Bus Creator10/5
  Demux29/4 -> Bus Creator6/8
  Demux9/10 -> Bus Creator2/42  "M/E Soot blower #26 Sol. VV"
  Demux2/15 -> Bus Creator1/31  "M/E Soot blower #7 Sol. VV"
  Demux18/7 -> Bus Creator7/23  "No.2 G/E Soot blower #11 Sol. VV"
  Demux8/16 -> Bus Creator2/32  "M/E Soot blower #16 Sol. VV"
  Demux11/1 -> Bus Creator3/1
  Demux27/1 -> Bus Creator3/5  "M/E Dosing urea control VV"
  Demux27/3 -> Bus Creator3/7  "Exh. gas flow (Burner Inlet)"
  Demux4/13 -> Bus Creator1/61  "M/E Soot blower #37 Sol. VV"
  Demux27/4 -> Bus Creator3/8
  Demux30/1 -> Bus Creator8/5
  Demux10/2 -> Bus Creator2/50  "M/E Soot blower #34 Sol. VV"
  Demux7/15 -> Bus Creator2/15
  Demux12/1 -> Bus Creator3/9  "Burner Setpoint"
  Demux10/1 -> Bus Creator2/49  "M/E Soot blower #33 Sol. VV"
  Demux23/8 -> Bus Creator12/8  "No.4 G/E RSV Setpoint"
  Demux10/11 -> Bus Creator2/59
  Demux8/1 -> Bus Creator2/17  "M/E Soot blower #1 Sol. VV"
  Demux21/5 -> Bus Creator9/21  "No.3 G/E Soot blower #9 Sol. VV"
  Structure Input1/1 -> Demux1/1
  Demux24/7 -> Bus Creator12/23  "No.4 G/E Soot blower #11 Sol. VV"
  Demux8/3 -> Bus Creator2/19  "M/E Soot blower #3 Sol. VV"
  Demux10/7 -> Bus Creator2/55
  Demux12/4 -> Bus Creator3/12  "Blower Setpoint"
  Bus Creator2/1 -> HP_DO/1
  Demux12/3 -> Bus Creator3/11  "M/E Load signal (To Burner)"
  Demux28/1 -> Bus Creator3/13  "M/E RTV Setpoint"
  Demux21/11 -> Bus Creator9/27
  Structure Input11/1 -> Demux10/1
  Demux9/7 -> Bus Creator2/39  "M/E Soot blower #23 Sol. VV"
  Demux10/12 -> Bus Creator2/60
  Demux25/3 -> Bus Creator11/3
  Demux9/1 -> Bus Creator2/33  "M/E Soot blower #17 Sol. VV"
  Demux10/15 -> Bus Creator2/63
  Demux10/13 -> Bus Creator2/61
  Bus Creator10/1 -> GE3_AO/1
  Demux7/11 -> Bus Creator2/11
  Demux7/5 -> Bus Creator2/5
  Demux7/12 -> Bus Creator2/12
  Demux24/13 -> Bus Creator12/29
  Demux9/11 -> Bus Creator2/43  "M/E Soot blower #27 Sol. VV"
  Demux7/6 -> Bus Creator2/6
  Demux32/4 -> Bus Creator11/8
  Demux8/5 -> Bus Creator2/21  "M/E Soot blower #5 Sol. VV"
  Demux9/4 -> Bus Creator2/36  "M/E Soot blower #20 Sol. VV"
  Demux10/4 -> Bus Creator2/52  "M/E Soot blower #36 Sol. VV"
  Demux9/8 -> Bus Creator2/40  "M/E Soot blower #24 Sol. VV"
  Demux23/15 -> Bus Creator12/15
  Demux10/3 -> Bus Creator2/51  "M/E Soot blower #35 Sol. VV"
  Bus Creator6/1 -> GE1_AO/1
  Demux24/8 -> Bus Creator12/24  "No.4 G/E Soot blower #12 Sol. VV"
  Demux10/10 -> Bus Creator2/58
  Demux32/1 -> Bus Creator11/5
  Demux25/4 -> Bus Creator11/4
  Demux16/1 -> Bus Creator6/1  "No.1 G/E Dosing urea control VV"
  Demux24/1 -> Bus Creator12/17  "No.4 G/E Soot blower #5 Sol. VV"
  Demux32/3 -> Bus Creator11/7
  Demux32/2 -> Bus Creator11/6
  Demux24/2 -> Bus Creator12/18  "No.4 G/E Soot blower #6 Sol. VV"
  Demux24/6 -> Bus Creator12/22  "No.4 G/E Soot blower #10 Sol. VV"
  Demux24/15 -> Bus Creator12/31
  Structure Input5/1 -> Demux4/1
  Demux24/11 -> Bus Creator12/27
  Bus Creator9/1 -> GE3_DO/1
  Demux24/12 -> Bus Creator12/28
  Demux24/14 -> Bus Creator12/30
  Demux24/10 -> Bus Creator12/26
  Demux23/10 -> Bus Creator12/10
  Demux30/4 -> Bus Creator8/8
  Structure Input21/1 -> Demux20/1
  Demux23/11 -> Bus Creator12/11
  Demux23/3 -> Bus Creator12/3  "No.4 G/E Dosing purging Sol. VV"
  Demux19/1 -> Bus Creator8/1  "No.2 G/E Dosing urea control VV"
  Demux23/4 -> Bus Creator12/4  "No.4 G/E Soot blower #1 Sol. VV"
  Demux23/7 -> Bus Creator12/7  "No.4 G/E Soot blower #4 Sol. VV"
  Demux16/3 -> Bus Creator6/3
  Demux19/4 -> Bus Creator8/4
  Demux18/1 -> Bus Creator7/17  "No.2 G/E Soot blower #5 Sol. VV"
  Demux18/2 -> Bus Creator7/18  "No.2 G/E Soot blower #6 Sol. VV"
  Demux21/15 -> Bus Creator9/31
  Demux18/3 -> Bus Creator7/19  "No.2 G/E Soot blower #7 Sol. VV"
  Demux18/14 -> Bus Creator7/30
  Demux18/16 -> Bus Creator7/32
  Bus Creator8/1 -> GE2_AO/1
  Demux15/8 -> Bus Creator5/24  "No.1 G/E Soot blower #12 Sol. VV"
  Demux18/15 -> Bus Creator7/31
  Demux17/15 -> Bus Creator7/15
  Demux21/14 -> Bus Creator9/30
  Demux19/3 -> Bus Creator8/3
  Demux19/2 -> Bus Creator8/2
  Demux3/1 -> Bus Creator1/33  "M/E Soot blower #9 Sol. VV"
  Demux15/5 -> Bus Creator5/21  "No.1 G/E Soot blower #9 Sol. VV"
  Demux15/2 -> Bus Creator5/18  "No.1 G/E Soot blower #6 Sol. VV"
  Demux20/15 -> Bus Creator9/15
  Demux20/2 -> Bus Creator9/2  "No.3 G/E Dosing air Sol. VV"
  Demux20/6 -> Bus Creator9/6  "No.3 G/E Soot blower #3 Sol. VV"
  Demux21/12 -> Bus Creator9/28
  Demux21/2 -> Bus Creator9/18  "No.3 G/E Soot blower #6 Sol. VV"
  Demux21/4 -> Bus Creator9/20  "No.3 G/E Soot blower #8 Sol. VV"
  Demux22/1 -> Bus Creator10/1  "No.3 G/E Dosing urea control VV"
  Demux16/4 -> Bus Creator6/4
  Demux29/3 -> Bus Creator6/7
  Demux29/1 -> Bus Creator6/5
  Demux2/7 -> Bus Creator1/23  "M/E ASV Setpoint"
  Demux2/14 -> Bus Creator1/30  "M/E Soot blower #6 Sol. VV"
  Bus Creator12/1 -> GE4_DO/1
  Bus Creator7/1 -> GE2_DO/1
  Demux13/2 -> Bus Creator13/2
  Demux13/3 -> Bus Creator13/3
  Bus Creator13/1 -> HP_AO/1
  Demux13/4 -> Bus Creator13/4
  Demux13/1 -> Bus Creator13/1
  Demux26/4 -> Bus Creator13/8
  Structure Input27/1 -> Demux13/1
  Demux26/1 -> Bus Creator13/5  "M/E Dosing urea control VV"
  Demux26/2 -> Bus Creator13/6
  Demux26/3 -> Bus Creator13/7
  Structure Input28/1 -> Demux27/1
  Structure Input29/1 -> Demux28/1
  Structure Input13/1 -> Demux12/1
  Structure Input14/1 -> Demux26/1
  Structure Input17/1 -> Demux29/1
  Structure Input30/1 -> Demux16/1
  Structure Input31/1 -> Demux19/1
  Structure Input20/1 -> Demux30/1
  Structure Input32/1 -> Demux22/1
  Structure Input23/1 -> Demux31/1
  Structure Input26/1 -> Demux32/1
  Structure Input33/1 -> Demux25/1
